simulink subsystem "ElectricalSystemArchitecture"  (R2023b)
settings: Solver=VariableStepAuto  StartTime=0.0  StopTime=10.0  RelTol=1e-3
undefined symbols (not defined in the file or in its folder): PlntDCDCVoltInit
settings Model: Creator=The MathWorks, Inc.  LastModifiedBy=Hp

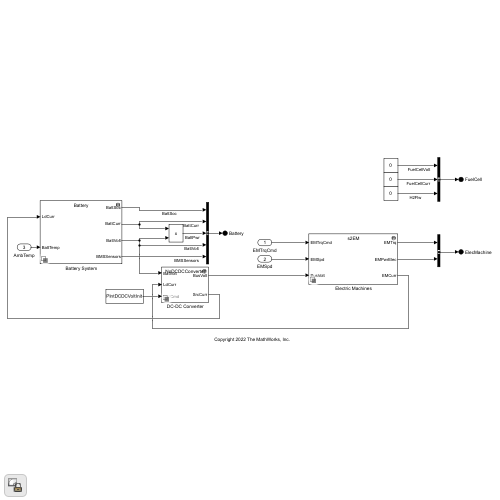
[thumbnail: Simulink's stored preview of the top-level diagram]
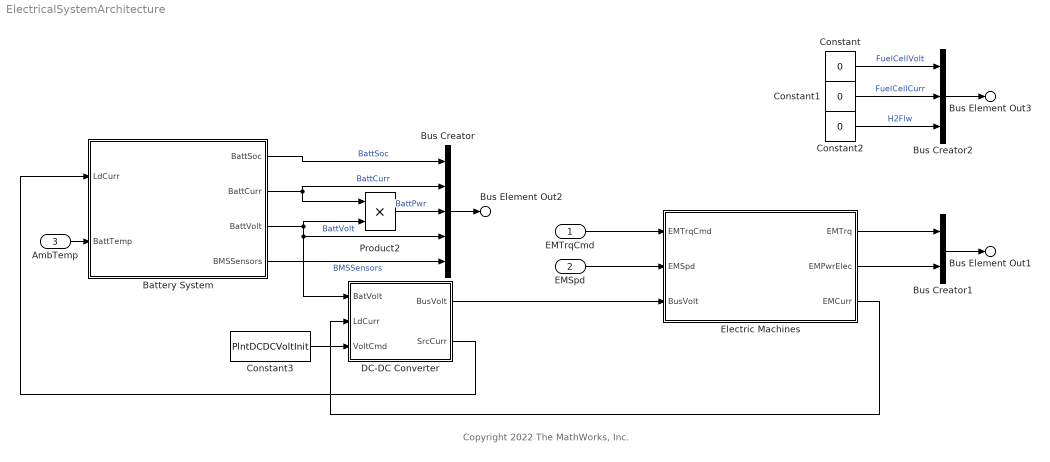
== system ElectricalSystemArchitecture ==
  note: Copyright 2022 The MathWorks, Inc.
  EMTrqCmd : Inport
  EMSpd : Inport  Port=2
  AmbTemp : Inport  Port=3
  Battery System : Subsystem  Variant=on  VariantChoicesSpecifier={'Battery'}  VariantControlMode=label  LabelModeActiveChoice=Battery
  Bus Creator : BusCreator  Inputs=5
  Bus Creator1 : BusCreator  Inputs=2
  Bus Creator2 : BusCreator  Inputs=3
  Constant : Constant  Value=0  SampleTime=-1
  Constant1 : Constant  Value=0  SampleTime=-1
  Constant2 : Constant  Value=0  SampleTime=-1
  Constant3 : Constant  Value=PlntDCDCVoltInit  SampleTime=-1
  DC-DC Converter : Subsystem  Variant=on  VariantChoicesSpecifier={'NoDCDCConverter'}  VariantControlMode=label  VariantControl=Choice  LabelModeActiveChoice=NoDCDCConverter
  Electric Machines : Subsystem  Variant=on  VariantChoicesSpecifier={'s2EM'}  VariantControlMode=label  VariantControl=Choice  LabelModeActiveChoice=s2EM
  Product2 : Product
  Bus Element Out2 : Outport  PortName=Battery
  Bus Element Out1 : Outport  Port=2  PortName=ElecMachine
  Bus Element Out3 : Outport  Port=3  PortName=FuelCell
  wires:
  AmbTemp/1 -> Battery System/2(BattTemp)
  Battery System/2(BattCurr) -> Product2/1, Bus Creator/2  "BattCurr"
  Battery System/1(BattSoc) -> Bus Creator/1  "BattSoc"
  Battery System/3(BattVolt) -> Product2/2, Bus Creator/4, DC-DC Converter/1(BatVolt)  "BattVolt"
  Product2/1 -> Bus Creator/3  "BattPwr"
  Bus Creator2/1 -> Bus Element Out3/1
  Bus Creator1/1 -> Bus Element Out1/1
  Constant/1 -> Bus Creator2/1  "FuelCellVolt"
  Constant1/1 -> Bus Creator2/2  "FuelCellCurr"
  Bus Creator/1 -> Bus Element Out2/1
  Constant2/1 -> Bus Creator2/3  "H2Flw"
  DC-DC Converter/2(SrcCurr) -> Battery System/1(LdCurr)
  Constant3/1 -> DC-DC Converter/3(VoltCmd)
  Battery System/4(BMSSensors) -> Bus Creator/5  "BMSSensors"
  EMTrqCmd/1 -> Electric Machines/1(EMTrqCmd)
  EMSpd/1 -> Electric Machines/2(EMSpd)
  DC-DC Converter/1(BusVolt) -> Electric Machines/3(BusVolt)
  Electric Machines/1(EMTrq) -> Bus Creator1/1
  Electric Machines/2(EMPwrElec) -> Bus Creator1/2
  Electric Machines/3(EMCurr) -> DC-DC Converter/2(LdCurr)

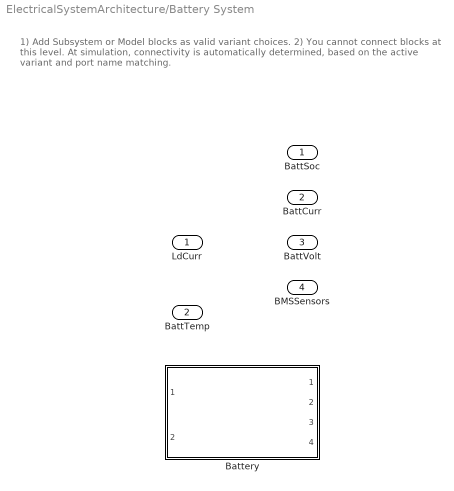
== system ElectricalSystemArchitecture/Battery System ==
  note: 1) Add Subsystem or Model blocks as valid variant choices.
      | 2) You cannot connect blocks at this level. At simulation, connectivity is automatically
      | determined, based on the active variant and port name matching.
  LdCurr : Inport
  BattTemp : Inport  Port=2
  Battery : Subsystem  VariantControl=Battery  ReferencedSubsystem=Battery
  BattSoc : Outport  VectorParamsAs1DForOutWhenUnconnected=off
  BattCurr : Outport  Port=2  VectorParamsAs1DForOutWhenUnconnected=off
  BattVolt : Outport  Port=3  VectorParamsAs1DForOutWhenUnconnected=off
  BMSSensors : Outport  Port=4  VectorParamsAs1DForOutWhenUnconnected=off

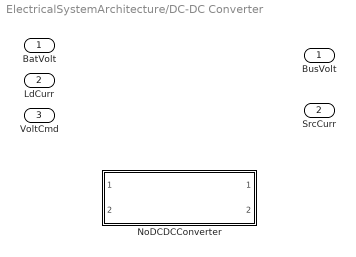
== system ElectricalSystemArchitecture/DC-DC Converter ==
  BatVolt : Inport
  LdCurr : Inport  Port=2
  VoltCmd : Inport  Port=3
  NoDCDCConverter : Subsystem  VariantControl=NoDCDCConverter  ReferencedSubsystem=NoDCDCConverter
  BusVolt : Outport
  SrcCurr : Outport  Port=2

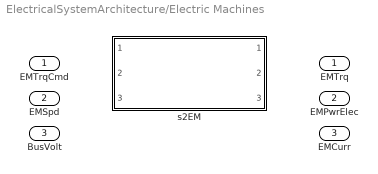
== system ElectricalSystemArchitecture/Electric Machines ==
  EMTrqCmd : Inport
  EMSpd : Inport  Port=2
  BusVolt : Inport  Port=3
  s2EM : Subsystem  VariantControl=s2EM  ReferencedSubsystem=s2EM
  EMTrq : Outport
  EMPwrElec : Outport  Port=2
  EMCurr : Outport  Port=3
